simulink model "n2k_parsing"  (Simulink 7.5)
settings: Solver=FixedStepDiscrete  SolverMode=SingleTasking  StartTime=0.0  StopTime=10.0  FixedStep=0.01  RelTol=1e-3
undefined symbols (not defined in the file): DisplayAirData, DisplayCourseAndSpeedData, DisplayDateData, DisplayLocationData, DisplayTimeData, DisplayWaterData, DisplayWindData, enqueueNumberText, GetAirData, GetCourseAndSpeedData, GetLocationData, GetTimeAndDateData, GetWaterData, GetWindData, Init_onlyOnce, Init_Reset, initCommunications, u1, u2, u3, y1
libraries: dsPICdrivers x19, uSimLib x4, simulink x2, ecan_dspic x1
settings Model: Creator=Bryant  LastModifiedBy=Bryant
settings OptimizationCC: InlineParams=on  OptimizeModelRefInitCode=on  LifeSpan=1
settings HardwareCC: ProdBitPerInt=16  ProdEndianess=LittleEndian  ProdWordSize=16  ProdHWDeviceType=16-bit Generic
settings RTWCC: SystemTargetFile=dspic.tlc  MakeCommand=make_CreateMPLAB  TemplateMakefile=dspic_pic30_gcc.tmf  PostCodeGenCommand=dsPIC_Compile()  Description=Embedded Target for Microchip dsPIC (real-time)  ProcessScript=dspic_make_rtw_hook
settings RTWCC: CustomSource=|
  | ../../../../../ECAN_dspic/CircularBuffer.c
  | ../../../../../ECAN_dspic/ecanFunctions.c
  | ../../clib/uart2.c
  | extra.c
  | ../../clib/nmea2000.c
settings CodeAppCC: IgnoreCustomStorageClasses=off
settings STFCustomTargetCC: IncludeMdlTerminateFcn=off  CombineOutputUpdateFcns=on  SuppressErrorStatus=on  ERTCustomFileBanners=on  SupportContinuousTime=off  SupportNonInlinedSFcns=off  SystemTargetFile=dspic.tlc
settings ERTTargetCC: MultiwordLength=2048  ParMdlRefBuildCompliant=off  CompOptLevelCompliant=off  IncludeMdlTerminateFcn=off  SuppressErrorStatus=on  ERTFirstTimeCompliant=off  ModelStepFunctionPrototypeControlCompliant=off  CPPClassGenCompliant=off  ExtModeMexFile=ext_serial_win32_comm  InlinedParameterPlacement=NonHierarchical  ERTSrcFileBannerTemplate=dsPIC_code_template.cgt  ERTHdrFileBannerTemplate=dsPIC_code_template.cgt  ERTDataSrcFileTemplate=dsPIC_code_template.cgt  ERTDataHdrFileTemplate=dsPIC_code_template.cgt  ERTCustomFileTemplate=dsPIC_main.tlc  ConvertIfToSwitch=off
settings CustomProperty: DataType=string  Value=C:\PROGRA~1\MATLAB\R2010a\bin\win64\gmake

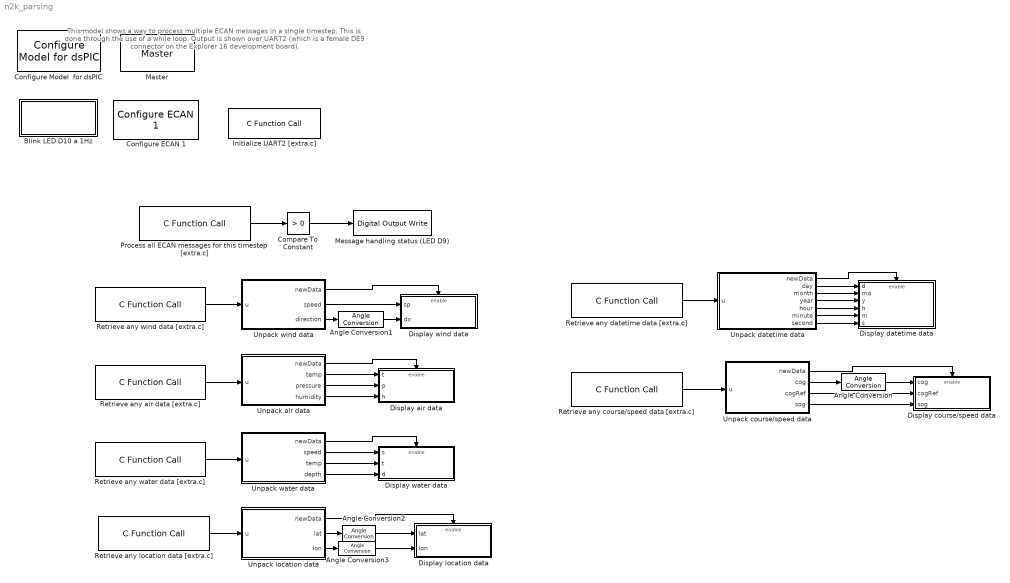
== system n2k_parsing ==
  note: This model shows a way to process multiple ECAN messages in a single timestep. This is done through the use of a while loop.
      | Output is shown over UART2 (which is a female DE9 connector on the Explorer 16 development board).
  Angle Conversion{,1..3} (4 alike) : uSimLib/Conversions/Angle Conversion  SystemSampleTime=-1  iu=rad  ou=deg
  Blink LED D10 a 1Hz : Subsystem
      mask Display: disp('blink');
  Compare To Constant : simulink/Logic and Bit Operations/Compare To Constant  SystemSampleTime=-1  relop=>  const=0  LogicOutDataTypeMode=boolean
  Configure ECAN 1 : ecan_dspic/Configure ECAN 1  SystemSampleTime=-1  frame_setting=on  mode=Normal  dma_rx_chan=2  dma_tx_chan=0  baud=250000  ps1=8  pd=5  ps2=6  sjw=4  tq=20  triple_sample=on  dma_buf_size=4 buffers  rx_bufs=[1]  tx_bufs=[0]  buf_0_tx_pri=Highest  buf_0_rte=No  buf_1_tx_pri=Highest  buf_1_rte=No  buf_2_tx_pri=Lowest  buf_2_rte=No  buf_3_tx_pri=Lowest  buf_3_rte=No  buf_4_tx_pri=Lowest  buf_4_rte=No  buf_5_tx_pri=Lowest  buf_5_rte=No  buf_6_tx_pri=Lowest  buf_6_rte=No  buf_7_tx_pri=Lowest  buf_7_rte=No  mask_0=0  mask_0_mide=Match std or ext  mask_1=0  mask_1_mide=Match std or ext  mask_2=0  mask_2_mide=Match std or ext  filters=[0]  filter_0=0  filter_0_mask=0  filter_0_exide=Match only extended  filter_0_buf=1  filter_1=hex2dec('401')  filter_1_mask=0  filter_1_exide=Match only standard  filter_1_buf=2  filter_2=hex2dec('402')  filter_2_mask=0  filter_2_exide=Match only standard  filter_2_buf=3  filter_3=0  filter_3_mask=0  filter_3_exide=Match only standard  filter_3_buf=0  filter_4=0  filter_4_mask=0  filter_4_exide=Match only standard  filter_4_buf=0  filter_5=0  filter_5_mask=0  filter_5_exide=Match only standard  filter_5_buf=0  filter_6=0  filter_6_mask=0  filter_6_exide=Match only standard  filter_6_buf=0  filter_7=0  filter_7_mask=0  filter_7_exide=Match only standard  filter_7_buf=0  filter_8=0  filter_8_mask=0  filter_8_exide=Match only standard  filter_8_buf=0  filter_9=0  filter_9_mask=<empty>  filter_9_exide=Match only standard  filter_9_buf=0  filter_10=0  filter_10_mask=0  filter_10_exide=Match only standard  filter_10_buf=0  filter_11=0  filter_11_mask=0  filter_11_exide=Match only standard  filter_11_buf=0  filter_12=0  filter_12_mask=0  filter_12_exide=Match only standard  filter_12_buf=0  filter_13=0  filter_13_mask=0  filter_13_exide=Match only standard  filter_13_buf=0  filter_14=0  filter_14_mask=0  filter_14_exide=Match only standard  filter_14_buf=0  filter_15=0  filter_15_mask=0  filter_15_exide=Match only standard  filter_15_buf=0
  Configure Model  for dsPIC : dsPICdrivers/Simulink Configuration/Configure Model  for dsPIC
  Display air data : Subsystem  TreatAsAtomicUnit=on
  Display course/speed data : Subsystem  TreatAsAtomicUnit=on
  Display datetime data : Subsystem  TreatAsAtomicUnit=on
  Display location data : Subsystem  TreatAsAtomicUnit=on
  Display water data : Subsystem  TreatAsAtomicUnit=on
  Display wind data : Subsystem  TreatAsAtomicUnit=on
  Initialize UART2 [extra.c] : dsPICdrivers/OTHERS/C Function Call  Tag=dsPIC_dsPIC_CFunctionCall  FctUpdate=None  fctName=enqueueNumberText  INPUT_SIZE=1  INPUT1=uint32  INPUT2=--  INPUT3=--  OUTPUT_SIZE=1  OUTPUT1=--  SampleTime=-1  InputType=[]  OutputType=[]  FctDeclaration=extern void enqueueNumberText();  FctCall=enqueueNumberText();  OrderingInOutPopup=None  FctStart=Start Function (Call once and only once)  FctStart_Name=initCommunications  FctStart_Declaration=inline extern void initCommunications();  FctStart_Call=initCommunications();  FctInit=None  FctInit_Name=Init_Reset  FctInit_Declaration=inline extern void Init_Reset();  FctInit_Call=Init_Reset();  PinDigitalInput=[]  PinDigitalOutput=[]  AnalogueInput=[]
  Master : dsPICdrivers/Master  Tag=dsPIC_MASTER  Priority=1  TimeStepType=Timer1  picType=33fJ256GP710  fcy=40000000  Quartz_33f=8e6  PLLActive_33f=on  fcyDesired_33f=40000000  tmr1="[8  49999  0]"  tmr1Info="Time Step : 0.01  ;   Error : 0%  PR1=49999"  tmr2345="[0  0  0  0  0  0  0  0]"  tmr2345cfg=[-1 -1 -1 -1 -1 -1 -1 -1]  IOautoConf=on  typePort="[ 0   0   0   0   0   0  10  10   0   0   0   0   0   0   0   0   0   0   0   0   0   0   0   0   0   0   0   0   0   0   0   0   0   0   0   0   0   0   0   0   0   0   0   0   0   0   0   0   0   0   0   0   0   0   0   0   0   0   0   0   0   0   0   0   0   0   0   0   0   0   0   0   0   0   0   0   0   0   0   0   0   0   0   0   0   0   0   0   0   0   0   0   0   0   0   0   0   0   0   0   0   0   0   0   0   0   0   0   0   0   0   0 ]"  TRIS="[ 65343  65535  65535  65535  65535  65535  65535 ]"  ADPCFG=12582912  MasterBusyPort=None  MasterOverloadPort=None  FOSC=Quartz (XT - HS)  ClockSwitchMonitor=Both disabled  TempProtection_33f=TEMP_ON  FPBOR=<empty>  PWRT=disable  MCLR=<empty>  ICD=ICS_PGD1  JTAGEN=JTAGEN_OFF  PowerSave=off  OverrideFcy=off  NewFcy=1e6  PR2345="[65535  65535  65535  65535  65535  65535  65535  65535]"
  Message handling status (LED D9) : dsPICdrivers/Digital I//O/Digital Output Write  Tag=dsPIC_Digital_Output  Priority=5  PORT=A  Pin=[6]  Simultaneous=off  OrderingInOutPopup=None
  Process all ECAN messages for this timestep [extra.c] : dsPICdrivers/OTHERS/C Function Call  Tag=dsPIC_dsPIC_CFunctionCall  FctUpdate=Output Function  fctName=processAllMessages  INPUT_SIZE=1  INPUT1=--  INPUT2=--  INPUT3=--  OUTPUT_SIZE=1  OUTPUT1=uint8  SampleTime=.01  InputType=[ ]  OutputType=[ 2 ]  FctDeclaration=extern uint8_T processAllMessages();  FctCall=%y1 = processAllMessages();  OrderingInOutPopup=None  FctStart=None  FctStart_Name=Init_onlyOnce  FctStart_Declaration=inline extern void Init_onlyOnce();  FctStart_Call=Init_onlyOnce();  FctInit=None  FctInit_Name=Init_Reset  FctInit_Declaration=inline extern void Init_Reset();  FctInit_Call=Init_Reset();  PinDigitalInput=[]  PinDigitalOutput=[]  AnalogueInput=[]
  Retrieve any air data [extra.c] : dsPICdrivers/OTHERS/C Function Call  Tag=dsPIC_dsPIC_CFunctionCall  FctUpdate=Output Function  fctName=GetAirData  INPUT_SIZE=1  INPUT1=--  INPUT2=--  INPUT3=--  OUTPUT_SIZE=13  OUTPUT1=uint8  SampleTime=.01  InputType=[ ]  OutputType=[ 2 ]  FctDeclaration=extern void GetAirData(uint8_T* y1);  FctCall=GetAirData(*%y1);  OrderingInOutPopup=None  FctStart=None  FctStart_Name=Init_onlyOnce  FctStart_Declaration=inline extern void Init_onlyOnce();  FctStart_Call=Init_onlyOnce();  FctInit=None  FctInit_Name=Init_Reset  FctInit_Declaration=inline extern void Init_Reset();  FctInit_Call=Init_Reset();  PinDigitalInput=[]  PinDigitalOutput=[]  AnalogueInput=[]
  Retrieve any course/speed data [extra.c] : dsPICdrivers/OTHERS/C Function Call  Tag=dsPIC_dsPIC_CFunctionCall  FctUpdate=Output Function  fctName=GetCourseAndSpeedData  INPUT_SIZE=1  INPUT1=--  INPUT2=--  INPUT3=--  OUTPUT_SIZE=10  OUTPUT1=uint8  SampleTime=.01  InputType=[ ]  OutputType=[ 2 ]  FctDeclaration=extern void GetCourseAndSpeedData(uint8_T* y1);  FctCall=GetCourseAndSpeedData(*%y1);  OrderingInOutPopup=None  FctStart=None  FctStart_Name=Init_onlyOnce  FctStart_Declaration=inline extern void Init_onlyOnce();  FctStart_Call=Init_onlyOnce();  FctInit=None  FctInit_Name=Init_Reset  FctInit_Declaration=inline extern void Init_Reset();  FctInit_Call=Init_Reset();  PinDigitalInput=[]  PinDigitalOutput=[]  AnalogueInput=[]
  Retrieve any datetime data [extra.c] : dsPICdrivers/OTHERS/C Function Call  Tag=dsPIC_dsPIC_CFunctionCall  FctUpdate=Output Function  fctName=GetTimeAndDateData  INPUT_SIZE=1  INPUT1=--  INPUT2=--  INPUT3=--  OUTPUT_SIZE=7  OUTPUT1=uint8  SampleTime=.01  InputType=[ ]  OutputType=[ 2 ]  FctDeclaration=extern void GetTimeAndDateData(uint8_T* y1);  FctCall=GetTimeAndDateData(*%y1);  OrderingInOutPopup=None  FctStart=None  FctStart_Name=Init_onlyOnce  FctStart_Declaration=inline extern void Init_onlyOnce();  FctStart_Call=Init_onlyOnce();  FctInit=None  FctInit_Name=Init_Reset  FctInit_Declaration=inline extern void Init_Reset();  FctInit_Call=Init_Reset();  PinDigitalInput=[]  PinDigitalOutput=[]  AnalogueInput=[]
  Retrieve any location data [extra.c] : dsPICdrivers/OTHERS/C Function Call  Tag=dsPIC_dsPIC_CFunctionCall  FctUpdate=Output Function  fctName=GetLocationData  INPUT_SIZE=1  INPUT1=--  INPUT2=--  INPUT3=--  OUTPUT_SIZE=9  OUTPUT1=uint8  SampleTime=.01  InputType=[ ]  OutputType=[ 2 ]  FctDeclaration=extern void GetLocationData(uint8_T* y1);  FctCall=GetLocationData(*%y1);  OrderingInOutPopup=None  FctStart=None  FctStart_Name=Init_onlyOnce  FctStart_Declaration=inline extern void Init_onlyOnce();  FctStart_Call=Init_onlyOnce();  FctInit=None  FctInit_Name=Init_Reset  FctInit_Declaration=inline extern void Init_Reset();  FctInit_Call=Init_Reset();  PinDigitalInput=[]  PinDigitalOutput=[]  AnalogueInput=[]
  Retrieve any water data [extra.c] : dsPICdrivers/OTHERS/C Function Call  Tag=dsPIC_dsPIC_CFunctionCall  FctUpdate=Output Function  fctName=GetWaterData  INPUT_SIZE=1  INPUT1=--  INPUT2=--  INPUT3=--  OUTPUT_SIZE=13  OUTPUT1=uint8  SampleTime=.01  InputType=[ ]  OutputType=[ 2 ]  FctDeclaration=extern void GetWaterData(uint8_T* y1);  FctCall=GetWaterData(*%y1);  OrderingInOutPopup=None  FctStart=None  FctStart_Name=Init_onlyOnce  FctStart_Declaration=inline extern void Init_onlyOnce();  FctStart_Call=Init_onlyOnce();  FctInit=None  FctInit_Name=Init_Reset  FctInit_Declaration=inline extern void Init_Reset();  FctInit_Call=Init_Reset();  PinDigitalInput=[]  PinDigitalOutput=[]  AnalogueInput=[]
  Retrieve any wind data [extra.c] : dsPICdrivers/OTHERS/C Function Call  Tag=dsPIC_dsPIC_CFunctionCall  FctUpdate=Output Function  fctName=GetWindData  INPUT_SIZE=1  INPUT1=--  INPUT2=--  INPUT3=--  OUTPUT_SIZE=9  OUTPUT1=uint8  SampleTime=.01  InputType=[ ]  OutputType=[ 2 ]  FctDeclaration=extern void GetWindData(uint8_T* y1);  FctCall=GetWindData(*%y1);  OrderingInOutPopup=None  FctStart=None  FctStart_Name=Init_onlyOnce  FctStart_Declaration=inline extern void Init_onlyOnce();  FctStart_Call=Init_onlyOnce();  FctInit=None  FctInit_Name=Init_Reset  FctInit_Declaration=inline extern void Init_Reset();  FctInit_Call=Init_Reset();  PinDigitalInput=[]  PinDigitalOutput=[]  AnalogueInput=[]
  Unpack air data : Stateflow chart  TreatAsAtomicUnit=on
  Unpack course/speed data : Stateflow chart  TreatAsAtomicUnit=on
  Unpack datetime data : Stateflow chart  TreatAsAtomicUnit=on
  Unpack location data : Stateflow chart  TreatAsAtomicUnit=on
  Unpack water data : Stateflow chart  TreatAsAtomicUnit=on
  Unpack wind data : Stateflow chart  TreatAsAtomicUnit=on
  wires:
  Process all ECAN messages for this timestep [extra.c]/1 -> Compare To Constant/1
  Compare To Constant/1 -> Message handling status (LED D9)/1
  Retrieve any wind data [extra.c]/1 -> Unpack wind data/1(u)
  Unpack wind data/1(newData) -> Display wind data/Enable
  Unpack wind data/3(direction) -> Angle Conversion1/1
  Unpack wind data/2(speed) -> Display wind data/1(sp)
  Retrieve any air data [extra.c]/1 -> Unpack air data/1(u)
  Unpack air data/1(newData) -> Display air data/Enable
  Unpack air data/3(pressure) -> Display air data/2(p)
  Unpack air data/2(temp) -> Display air data/1(t)
  Unpack air data/4(humidity) -> Display air data/3(h)
  Retrieve any water data [extra.c]/1 -> Unpack water data/1(u)
  Unpack water data/1(newData) -> Display water data/Enable
  Unpack water data/3(temp) -> Display water data/2(t)
  Unpack water data/4(depth) -> Display water data/3(d)
  Unpack water data/2(speed) -> Display water data/1(s)
  Retrieve any location data [extra.c]/1 -> Unpack location data/1(u)
  Unpack location data/1(newData) -> Display location data/Enable
  Unpack location data/3(lon) -> Angle Conversion3/1
  Unpack location data/2(lat) -> Angle Conversion2/1
  Retrieve any datetime data [extra.c]/1 -> Unpack datetime data/1(u)
  Unpack datetime data/1(newData) -> Display datetime data/Enable
  Unpack datetime data/2(day) -> Display datetime data/1(d)
  Unpack datetime data/3(month) -> Display datetime data/2(mo)
  Unpack datetime data/4(year) -> Display datetime data/3(y)
  Unpack datetime data/5(hour) -> Display datetime data/4(h)
  Unpack datetime data/6(minute) -> Display datetime data/5(m)
  Unpack datetime data/7(second) -> Display datetime data/6(s)
  Retrieve any course/speed data [extra.c]/1 -> Unpack course/speed data/1(u)
  Unpack course/speed data/1(newData) -> Display course/speed data/Enable
  Unpack course/speed data/3(cogRef) -> Display course/speed data/2(cogRef)
  Unpack course/speed data/2(cog) -> Angle Conversion/1
  Unpack course/speed data/4(sog) -> Display course/speed data/3(sog)
  Angle Conversion/1 -> Display course/speed data/1(cog)
  Angle Conversion1/1 -> Display wind data/2(dir)
  Angle Conversion2/1 -> Display location data/1(lat)
  Angle Conversion3/1 -> Display location data/2(lon)

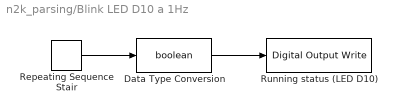
== system n2k_parsing/Blink LED D10 a 1Hz ==
  Data Type Conversion : DataTypeConversion  OutDataTypeMode=boolean  OutDataType=sfix(16)  OutScaling=2^0  OutDataTypeStr=boolean  RndMeth=Simplest
  Repeating Sequence Stair : simulink/Sources/Repeating Sequence Stair  SystemSampleTime=-1  OutValues=[1 0]  tsamp=1  OutMin=[]  OutMax=[]  OutDataTypeStr=double  OutputDataTypeScalingMode=double  OutDataType=fixdt(0,8)  ConRadixGroup=Best Precision: Vector-wise  OutScaling=2^-12
  Running status (LED D10) : dsPICdrivers/Digital I//O/Digital Output Write  Tag=dsPIC_Digital_Output  Priority=5  PORT=A  Pin=[7]  Simultaneous=off  OrderingInOutPopup=None
  wires:
  Repeating Sequence Stair/1 -> Data Type Conversion/1
  Data Type Conversion/1 -> Running status (LED D10)/1

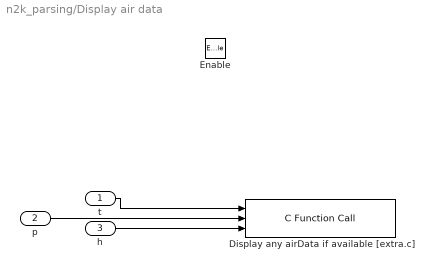
== system n2k_parsing/Display air data ==
  t : Inport  OutDataType=fixdt(1, 16)  OutScaling=2^0
  p : Inport  Port=2  OutDataType=fixdt(1, 16)  OutScaling=2^0
  h : Inport  Port=3  OutDataType=fixdt(1, 16)  OutScaling=2^0
  Enable : EnablePort
  Display any airData if available [extra.c] : dsPICdrivers/OTHERS/C Function Call  Tag=dsPIC_dsPIC_CFunctionCall  FctUpdate=Output Function  fctName=DisplayAirData  INPUT_SIZE=1  INPUT1=real32  INPUT2=real32  INPUT3=real32  OUTPUT_SIZE=1  OUTPUT1=--  SampleTime=.01  InputType=[ 7 7 7 ]  OutputType=[ ]  FctDeclaration=extern void DisplayAirData(real32_T u1, real32_T u2, real32_T u3);  FctCall=DisplayAirData(%u1, %u2, %u3);  OrderingInOutPopup=None  FctStart=None  FctStart_Name=Init_onlyOnce  FctStart_Declaration=inline extern void Init_onlyOnce();  FctStart_Call=Init_onlyOnce();  FctInit=None  FctInit_Name=Init_Reset  FctInit_Declaration=inline extern void Init_Reset();  FctInit_Call=Init_Reset();  PinDigitalInput=[]  PinDigitalOutput=[]  AnalogueInput=[]
  wires:
  t/1 -> Display any airData if available [extra.c]/1
  p/1 -> Display any airData if available [extra.c]/2
  h/1 -> Display any airData if available [extra.c]/3

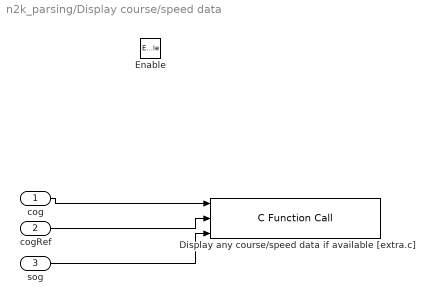
== system n2k_parsing/Display course/speed data ==
  cog : Inport  OutDataType=fixdt(1, 16)  OutScaling=2^0
  cogRef : Inport  Port=2  OutDataType=fixdt(1, 16)  OutScaling=2^0
  sog : Inport  Port=3  OutDataType=fixdt(1, 16)  OutScaling=2^0
  Enable : EnablePort
  Display any course/speed data if available [extra.c] : dsPICdrivers/OTHERS/C Function Call  Tag=dsPIC_dsPIC_CFunctionCall  FctUpdate=Output Function  fctName=DisplayCourseAndSpeedData  INPUT_SIZE=1  INPUT1=real32  INPUT2=uint8  INPUT3=real32  OUTPUT_SIZE=1  OUTPUT1=--  SampleTime=.01  InputType=[ 7 2 7 ]  OutputType=[ ]  FctDeclaration=extern void DisplayCourseAndSpeedData(real32_T u1, uint8_T u2, real32_T u3);  FctCall=DisplayCourseAndSpeedData(%u1, %u2, %u3);  OrderingInOutPopup=None  FctStart=None  FctStart_Name=Init_onlyOnce  FctStart_Declaration=inline extern void Init_onlyOnce();  FctStart_Call=Init_onlyOnce();  FctInit=None  FctInit_Name=Init_Reset  FctInit_Declaration=inline extern void Init_Reset();  FctInit_Call=Init_Reset();  PinDigitalInput=[]  PinDigitalOutput=[]  AnalogueInput=[]
  wires:
  cog/1 -> Display any course/speed data if available [extra.c]/1
  cogRef/1 -> Display any course/speed data if available [extra.c]/2
  sog/1 -> Display any course/speed data if available [extra.c]/3

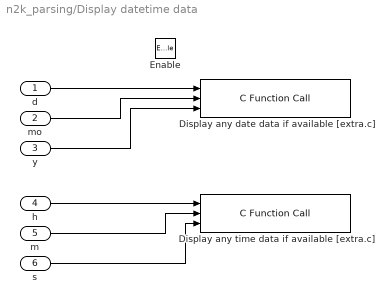
== system n2k_parsing/Display datetime data ==
  d : Inport  OutDataType=fixdt(1, 16)  OutScaling=2^0
  mo : Inport  Port=2  OutDataType=fixdt(1, 16)  OutScaling=2^0
  y : Inport  Port=3  OutDataType=fixdt(1, 16)  OutScaling=2^0
  h : Inport  Port=4  OutDataType=fixdt(1, 16)  OutScaling=2^0
  m : Inport  Port=5  OutDataType=fixdt(1, 16)  OutScaling=2^0
  s : Inport  Port=6  OutDataType=fixdt(1, 16)  OutScaling=2^0
  Enable : EnablePort
  Display any date data if available [extra.c] : dsPICdrivers/OTHERS/C Function Call  Tag=dsPIC_dsPIC_CFunctionCall  FctUpdate=Output Function  fctName=DisplayDateData  INPUT_SIZE=1  INPUT1=uint8  INPUT2=uint8  INPUT3=uint8  OUTPUT_SIZE=1  OUTPUT1=--  SampleTime=.01  InputType=[ 2 2 2 ]  OutputType=[ ]  FctDeclaration=extern void DisplayDateData(uint8_T u1, uint8_T u2, uint8_T u3);  FctCall=DisplayDateData(%u1, %u2, %u3);  OrderingInOutPopup=None  FctStart=None  FctStart_Name=Init_onlyOnce  FctStart_Declaration=inline extern void Init_onlyOnce();  FctStart_Call=Init_onlyOnce();  FctInit=None  FctInit_Name=Init_Reset  FctInit_Declaration=inline extern void Init_Reset();  FctInit_Call=Init_Reset();  PinDigitalInput=[]  PinDigitalOutput=[]  AnalogueInput=[]
  Display any time data if available [extra.c] : dsPICdrivers/OTHERS/C Function Call  Tag=dsPIC_dsPIC_CFunctionCall  FctUpdate=Output Function  fctName=DisplayTimeData  INPUT_SIZE=1  INPUT1=uint8  INPUT2=uint8  INPUT3=uint8  OUTPUT_SIZE=1  OUTPUT1=--  SampleTime=.01  InputType=[ 2 2 2 ]  OutputType=[ ]  FctDeclaration=extern void DisplayTimeData(uint8_T u1, uint8_T u2, uint8_T u3);  FctCall=DisplayTimeData(%u1, %u2, %u3);  OrderingInOutPopup=None  FctStart=None  FctStart_Name=Init_onlyOnce  FctStart_Declaration=inline extern void Init_onlyOnce();  FctStart_Call=Init_onlyOnce();  FctInit=None  FctInit_Name=Init_Reset  FctInit_Declaration=inline extern void Init_Reset();  FctInit_Call=Init_Reset();  PinDigitalInput=[]  PinDigitalOutput=[]  AnalogueInput=[]
  wires:
  h/1 -> Display any time data if available [extra.c]/1
  m/1 -> Display any time data if available [extra.c]/2
  s/1 -> Display any time data if available [extra.c]/3
  d/1 -> Display any date data if available [extra.c]/1
  mo/1 -> Display any date data if available [extra.c]/2
  y/1 -> Display any date data if available [extra.c]/3

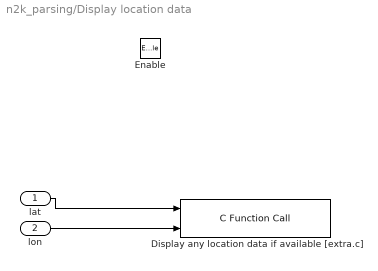
== system n2k_parsing/Display location data ==
  lat : Inport  OutDataType=fixdt(1, 16)  OutScaling=2^0
  lon : Inport  Port=2  OutDataType=fixdt(1, 16)  OutScaling=2^0
  Enable : EnablePort
  Display any location data if available [extra.c] : dsPICdrivers/OTHERS/C Function Call  Tag=dsPIC_dsPIC_CFunctionCall  FctUpdate=Output Function  fctName=DisplayLocationData  INPUT_SIZE=1  INPUT1=real32  INPUT2=real32  INPUT3=--  OUTPUT_SIZE=1  OUTPUT1=--  SampleTime=.01  InputType=[ 7 7 ]  OutputType=[ ]  FctDeclaration=extern void DisplayLocationData(real32_T u1, real32_T u2);  FctCall=DisplayLocationData(%u1, %u2);  OrderingInOutPopup=None  FctStart=None  FctStart_Name=Init_onlyOnce  FctStart_Declaration=inline extern void Init_onlyOnce();  FctStart_Call=Init_onlyOnce();  FctInit=None  FctInit_Name=Init_Reset  FctInit_Declaration=inline extern void Init_Reset();  FctInit_Call=Init_Reset();  PinDigitalInput=[]  PinDigitalOutput=[]  AnalogueInput=[]
  wires:
  lat/1 -> Display any location data if available [extra.c]/1
  lon/1 -> Display any location data if available [extra.c]/2

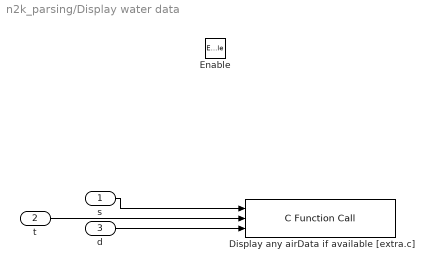
== system n2k_parsing/Display water data ==
  s : Inport  OutDataType=fixdt(1, 16)  OutScaling=2^0
  t : Inport  Port=2  OutDataType=fixdt(1, 16)  OutScaling=2^0
  d : Inport  Port=3  OutDataType=fixdt(1, 16)  OutScaling=2^0
  Enable : EnablePort
  Display any airData if available [extra.c] : dsPICdrivers/OTHERS/C Function Call  Tag=dsPIC_dsPIC_CFunctionCall  FctUpdate=Output Function  fctName=DisplayWaterData  INPUT_SIZE=1  INPUT1=real32  INPUT2=real32  INPUT3=real32  OUTPUT_SIZE=1  OUTPUT1=--  SampleTime=.01  InputType=[ 7 7 7 ]  OutputType=[ ]  FctDeclaration=extern void DisplayWaterData(real32_T u1, real32_T u2, real32_T u3);  FctCall=DisplayWaterData(%u1, %u2, %u3);  OrderingInOutPopup=None  FctStart=None  FctStart_Name=Init_onlyOnce  FctStart_Declaration=inline extern void Init_onlyOnce();  FctStart_Call=Init_onlyOnce();  FctInit=None  FctInit_Name=Init_Reset  FctInit_Declaration=inline extern void Init_Reset();  FctInit_Call=Init_Reset();  PinDigitalInput=[]  PinDigitalOutput=[]  AnalogueInput=[]
  wires:
  s/1 -> Display any airData if available [extra.c]/1
  t/1 -> Display any airData if available [extra.c]/2
  d/1 -> Display any airData if available [extra.c]/3

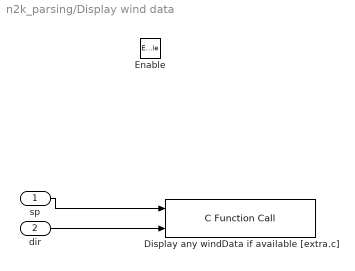
== system n2k_parsing/Display wind data ==
  sp : Inport  OutDataType=fixdt(1, 16)  OutScaling=2^0
  dir : Inport  Port=2  OutDataType=fixdt(1, 16)  OutScaling=2^0
  Enable : EnablePort
  Display any windData if available [extra.c] : dsPICdrivers/OTHERS/C Function Call  Tag=dsPIC_dsPIC_CFunctionCall  FctUpdate=Output Function  fctName=DisplayWindData  INPUT_SIZE=1  INPUT1=real32  INPUT2=real32  INPUT3=--  OUTPUT_SIZE=1  OUTPUT1=--  SampleTime=.01  InputType=[ 7 7 ]  OutputType=[ ]  FctDeclaration=extern void DisplayWindData(real32_T u1, real32_T u2);  FctCall=DisplayWindData(%u1, %u2);  OrderingInOutPopup=None  FctStart=None  FctStart_Name=Init_onlyOnce  FctStart_Declaration=inline extern void Init_onlyOnce();  FctStart_Call=Init_onlyOnce();  FctInit=None  FctInit_Name=Init_Reset  FctInit_Declaration=inline extern void Init_Reset();  FctInit_Call=Init_Reset();  PinDigitalInput=[]  PinDigitalOutput=[]  AnalogueInput=[]
  wires:
  sp/1 -> Display any windData if available [extra.c]/1
  dir/1 -> Display any windData if available [extra.c]/2

== matlab function Unpack air data ==
  data: newData output double; u input uint8; temp output double; pressure output double; humidity output double
function [newData, temp, pressure, humidity] = unpack(u)
%#eml

temp = typecast(u(1:4), 'single');
pressure = typecast(u(5:8), 'single');
humidity = typecast(u(9:12), 'single');
newData = u(13);

== matlab function Unpack water data ==
  data: newData output double; speed output double; u input uint8; temp output double; depth output double
function [newData, speed, temp, depth] = unpack(u)
%#eml

speed = typecast(u(1:4), 'single');
temp = typecast(u(5:8), 'single');
depth = typecast(u(9:12), 'single');
newData = u(13);

== matlab function Unpack location data ==
  data: newData output double; lat output double; u input uint8; lon output double
function [newData, lat, lon] = unpack(u)
%#eml

lat = typecast(u(1:4), 'single');
lon = typecast(u(5:8), 'single');
newData = u(9);

== matlab function Unpack datetime data ==
  data: newData output double; u input uint8; day output double; month output double; year output double; hour output double; minute output double; second output double
function [newData, day, month, year, hour, minute, second] = unpack(u)
%#eml

day = u(1);
month = u(2);
year = u(3);
hour = u(4);
minute = u(5);
second = u(6);
newData = u(7);

== matlab function Unpack course/speed data ==
  data: newData output double; cog output double; u input uint8; cogRef output double; sog output double
function [newData, cog, cogRef, sog] = unpack(u)
%#eml

cog = typecast(u(1:4), 'single');
cogRef = u(5);
sog = typecast(u(6:9), 'single');
newData = u(10);

== matlab function Unpack wind data ==
  data: newData output double; u input uint8; speed output double; direction output double
function [newData, speed, direction] = unpack(u)
%#eml

speed = typecast(u(1:4), 'single');
direction = typecast(u(5:8), 'single');
newData = u(9);
